simulink model "quadcopter_swarm_Perron_quaternion"  (R2023b)
settings: Solver=ode3  StartTime=0  StopTime=inf  FixedStep=0.005  RelTol=1e-3  EnableMultiTasking=on
values from neighbouring files (symbols this model uses):
  epsilon = 0.24975    [1nrx_dot.mat]    (also in 1nrxdrones_dot.mat; collision_avoidance_POS.mat; collision_avoidance_headonfix_POS.mat; collision_test.mat)
  F_e_g = [0 0 39.28]    [1nrx_dot.mat]    (also in 1nrxdrones_dot.mat; collision_avoidance_POS.mat; collision_avoidance_headonfix_POS.mat; collision_test.mat)
  g = 9.82    [1nrx_dot.mat]    (also in 1nrxdrones_dot.mat; collision_avoidance_POS.mat; collision_avoidance_headonfix_POS.mat; collision_test.mat)
  I_C = [0.5  0  0; 0  0.5  0; 0  0  1]    [1nrx_dot.mat]    (also in 1nrxdrones_dot.mat; collision_avoidance_POS.mat; collision_avoidance_headonfix_POS.mat; collision_test.mat)
  L = [4 -1 -1 -1 -1 0 -1 4 -1 -1 -1 0 ... (36 elements, 6x6)]    [1nrx_dot.mat]    (also in 1nrxdrones_dot.mat; collision_avoidance_POS.mat; collision_avoidance_headonfix_POS.mat; collision_test.mat)
  m = 4    [1nrx_dot.mat]    (also in 1nrxdrones_dot.mat; collision_avoidance_POS.mat; collision_avoidance_headonfix_POS.mat; collision_test.mat)
  M_RB = [4 0 0 0 0 0 0 4 0 0 0 0 ... (36 elements, 6x6)]    [1nrx_dot.mat]    (also in 1nrxdrones_dot.mat; collision_avoidance_POS.mat; collision_avoidance_headonfix_POS.mat; collision_test.mat)
  p_0 = [5  10; 5  -5; -8  5; 5  -13; 8  8; 0  0]    [1nrx_dot.mat]    (also in 1nrxdrones_dot.mat; collision_avoidance_POS.mat; collision_avoidance_headonfix_POS.mat; collision_test.mat)
  p_d = [1  0; 4  0; -2  0; 7  0; 9  0; 0  0]    [1nrx_dot.mat]    (also in 1nrxdrones_dot.mat; collision_avoidance_POS.mat; collision_avoidance_headonfix_POS.mat; collision_test.mat)
  V = [1 2 3 4 5 6]    [1nrx_dot.mat]    (also in 1nrxdrones_dot.mat; collision_avoidance_POS.mat; collision_avoidance_headonfix_POS.mat; collision_test.mat)
undefined symbols (not defined in the file or in its folder): PID_angle_max, PID_inner_max, PID_outer_max, PID_thrust_max
libraries: slpidlib x24, simulink_extras x20, dspsigops x15, sharedtransform x13, aerolibutil x11, dspindex x4, sharedutil x1, vrlib x1
(part 5 of 5)

== system quadcopter_swarm_Perron_quaternion/Master drone/Formatting/Euler to VR/Quaternion Normalization1 ==
  e0 : Inport
  1/2 : Gain  Gain=1/2  SaturateOnIntegerOverflow=on  OutDataTypeStr=Inherit: Same as input  ParamDataTypeStr=Inherit: Same as input
  Demux : Demux  Outputs=[1 3]
      settings: DisplayOption=none
  Mux : Mux  Inputs=2
  Product : Product  InputSameDT=on  SaturateOnIntegerOverflow=on  OutDataTypeStr=Inherit: Same as first input
  Trigonometric Function : Trigonometry
  Trigonometric Function1 : Trigonometry  Operator=cos
  e0_norm : Outport  VectorParamsAs1DForOutWhenUnconnected=off
  wires:
  e0/1 -> Demux/1
  1/2/1 -> Trigonometric Function/1, Trigonometric Function1/1
  Trigonometric Function/1 -> Product/1
  Product/1 -> Mux/2
  Mux/1 -> e0_norm/1
  Demux/1 -> 1/2/1
  Demux/2 -> Product/2
  Trigonometric Function1/1 -> Mux/1

== system quadcopter_swarm_Perron_quaternion/Master drone/Formatting/Euler to VR/Quaternion Normalization2 ==
  e0 : Inport
  1/2 : Gain  Gain=1/2  SaturateOnIntegerOverflow=on  OutDataTypeStr=Inherit: Same as input  ParamDataTypeStr=Inherit: Same as input
  Demux : Demux  Outputs=[1 3]
      settings: DisplayOption=none
  Mux : Mux  Inputs=2
  Product : Product  InputSameDT=on  SaturateOnIntegerOverflow=on  OutDataTypeStr=Inherit: Same as first input
  Trigonometric Function : Trigonometry
  Trigonometric Function1 : Trigonometry  Operator=cos
  e0_norm : Outport  VectorParamsAs1DForOutWhenUnconnected=off
  wires:
  Trigonometric Function1/1 -> Mux/1
  Demux/2 -> Product/2
  Demux/1 -> 1/2/1
  Mux/1 -> e0_norm/1
  Product/1 -> Mux/2
  Trigonometric Function/1 -> Product/1
  1/2/1 -> Trigonometric Function1/1, Trigonometric Function/1
  e0/1 -> Demux/1

== system quadcopter_swarm_Perron_quaternion/Master drone/Quadcopter model Euler/Gravity/euler_to_rotation ==
  eta_euler : Inport
  Rotation Angles to Direction Cosine Matrix : sharedtransform/Rotation Angles to Direction Cosine Matrix  rotationOrder=XYZ  aMode=aMode
  Selector : Selector  InputPortWidth=6  IndexOptions=Index vector (dialog)  Indices=4:6  OutputSizes=1
  R_e_b : Outport
  wires:
  Selector/1 -> Rotation Angles to Direction Cosine Matrix/1  "Theta_0"
  eta_euler/1 -> Selector/1
  Rotation Angles to Direction Cosine Matrix/1 -> R_e_b/1

== system quadcopter_swarm_Perron_quaternion/Master drone2/Formatting/Euler to VR/Axis Angle Vector ==
  e0 : Inport
  2 : Gain  Gain=2  SaturateOnIntegerOverflow=on  OutDataTypeStr=Inherit: Same as input  ParamDataTypeStr=Inherit: Same as input
  Constant : Constant  Value=1e-6
  Demux : Demux  Outputs=[1 3 ]
      settings: DisplayOption=none
  Mux : Mux  Inputs=2
  Product : Product  Inputs=*/  InputSameDT=on  SaturateOnIntegerOverflow=on  OutDataTypeStr=Inherit: Same as first input
  Switch : Switch  Criteria=u2 ~= 0  SaturateOnIntegerOverflow=off  InputSameDT=off
  Trigonometric Function : Trigonometry
  Trigonometric Function2 : Trigonometry  Operator=acos
  e0_norm : Outport  VectorParamsAs1DForOutWhenUnconnected=off
  wires:
  Demux/1 -> Trigonometric Function2/1
  Demux/2 -> Product/1
  Mux/1 -> e0_norm/1
  Product/1 -> Mux/1
  2/1 -> Mux/2
  Trigonometric Function/1 -> Switch/1, Switch/2
  Trigonometric Function2/1 -> Trigonometric Function/1, 2/1
  e0/1 -> Demux/1
  Constant/1 -> Switch/3
  Switch/1 -> Product/2

== system quadcopter_swarm_Perron_quaternion/Master drone2/Formatting/Euler to VR/Quaternion Normalization ==
  e0 : Inport
  1/2 : Gain  Gain=1/2  SaturateOnIntegerOverflow=on  OutDataTypeStr=Inherit: Same as input  ParamDataTypeStr=Inherit: Same as input
  Demux : Demux  Outputs=[1 3]
      settings: DisplayOption=none
  Mux : Mux  Inputs=2
  Product : Product  InputSameDT=on  SaturateOnIntegerOverflow=on  OutDataTypeStr=Inherit: Same as first input
  Trigonometric Function : Trigonometry
  Trigonometric Function1 : Trigonometry  Operator=cos
  e0_norm : Outport  VectorParamsAs1DForOutWhenUnconnected=off
  wires:
  Trigonometric Function1/1 -> Mux/1
  Demux/2 -> Product/2
  Demux/1 -> 1/2/1
  Mux/1 -> e0_norm/1
  Product/1 -> Mux/2
  Trigonometric Function/1 -> Product/1
  1/2/1 -> Trigonometric Function1/1, Trigonometric Function/1
  e0/1 -> Demux/1

== system quadcopter_swarm_Perron_quaternion/Master drone2/Formatting/Euler to VR/Quaternion Normalization1 ==
  e0 : Inport
  1/2 : Gain  Gain=1/2  SaturateOnIntegerOverflow=on  OutDataTypeStr=Inherit: Same as input  ParamDataTypeStr=Inherit: Same as input
  Demux : Demux  Outputs=[1 3]
      settings: DisplayOption=none
  Mux : Mux  Inputs=2
  Product : Product  InputSameDT=on  SaturateOnIntegerOverflow=on  OutDataTypeStr=Inherit: Same as first input
  Trigonometric Function : Trigonometry
  Trigonometric Function1 : Trigonometry  Operator=cos
  e0_norm : Outport  VectorParamsAs1DForOutWhenUnconnected=off
  wires:
  e0/1 -> Demux/1
  1/2/1 -> Trigonometric Function/1, Trigonometric Function1/1
  Trigonometric Function/1 -> Product/1
  Product/1 -> Mux/2
  Mux/1 -> e0_norm/1
  Demux/1 -> 1/2/1
  Demux/2 -> Product/2
  Trigonometric Function1/1 -> Mux/1

== system quadcopter_swarm_Perron_quaternion/Master drone2/Formatting/Euler to VR/Quaternion Normalization2 ==
  e0 : Inport
  1/2 : Gain  Gain=1/2  SaturateOnIntegerOverflow=on  OutDataTypeStr=Inherit: Same as input  ParamDataTypeStr=Inherit: Same as input
  Demux : Demux  Outputs=[1 3]
      settings: DisplayOption=none
  Mux : Mux  Inputs=2
  Product : Product  InputSameDT=on  SaturateOnIntegerOverflow=on  OutDataTypeStr=Inherit: Same as first input
  Trigonometric Function : Trigonometry
  Trigonometric Function1 : Trigonometry  Operator=cos
  e0_norm : Outport  VectorParamsAs1DForOutWhenUnconnected=off
  wires:
  Trigonometric Function1/1 -> Mux/1
  Demux/2 -> Product/2
  Demux/1 -> 1/2/1
  Mux/1 -> e0_norm/1
  Product/1 -> Mux/2
  Trigonometric Function/1 -> Product/1
  1/2/1 -> Trigonometric Function1/1, Trigonometric Function/1
  e0/1 -> Demux/1

== system quadcopter_swarm_Perron_quaternion/Master drone2/Quadcopter model Euler/Gravity/euler_to_rotation ==
  eta_euler : Inport
  Rotation Angles to Direction Cosine Matrix : sharedtransform/Rotation Angles to Direction Cosine Matrix  rotationOrder=XYZ  aMode=aMode
  Selector : Selector  InputPortWidth=6  IndexOptions=Index vector (dialog)  Indices=4:6  OutputSizes=1
  R_e_b : Outport
  wires:
  Selector/1 -> Rotation Angles to Direction Cosine Matrix/1  "Theta_0"
  eta_euler/1 -> Selector/1
  Rotation Angles to Direction Cosine Matrix/1 -> R_e_b/1

== system quadcopter_swarm_Perron_quaternion/Master drone3/Formatting/Euler to VR/Axis Angle Vector ==
  e0 : Inport
  2 : Gain  Gain=2  SaturateOnIntegerOverflow=on  OutDataTypeStr=Inherit: Same as input  ParamDataTypeStr=Inherit: Same as input
  Constant : Constant  Value=1e-6
  Demux : Demux  Outputs=[1 3 ]
      settings: DisplayOption=none
  Mux : Mux  Inputs=2
  Product : Product  Inputs=*/  InputSameDT=on  SaturateOnIntegerOverflow=on  OutDataTypeStr=Inherit: Same as first input
  Switch : Switch  Criteria=u2 ~= 0  SaturateOnIntegerOverflow=off  InputSameDT=off
  Trigonometric Function : Trigonometry
  Trigonometric Function2 : Trigonometry  Operator=acos
  e0_norm : Outport  VectorParamsAs1DForOutWhenUnconnected=off
  wires:
  Demux/1 -> Trigonometric Function2/1
  Demux/2 -> Product/1
  Mux/1 -> e0_norm/1
  Product/1 -> Mux/1
  2/1 -> Mux/2
  Trigonometric Function/1 -> Switch/1, Switch/2
  Trigonometric Function2/1 -> Trigonometric Function/1, 2/1
  e0/1 -> Demux/1
  Constant/1 -> Switch/3
  Switch/1 -> Product/2

== system quadcopter_swarm_Perron_quaternion/Master drone3/Formatting/Euler to VR/Quaternion Normalization ==
  e0 : Inport
  1/2 : Gain  Gain=1/2  SaturateOnIntegerOverflow=on  OutDataTypeStr=Inherit: Same as input  ParamDataTypeStr=Inherit: Same as input
  Demux : Demux  Outputs=[1 3]
      settings: DisplayOption=none
  Mux : Mux  Inputs=2
  Product : Product  InputSameDT=on  SaturateOnIntegerOverflow=on  OutDataTypeStr=Inherit: Same as first input
  Trigonometric Function : Trigonometry
  Trigonometric Function1 : Trigonometry  Operator=cos
  e0_norm : Outport  VectorParamsAs1DForOutWhenUnconnected=off
  wires:
  Trigonometric Function1/1 -> Mux/1
  Demux/2 -> Product/2
  Demux/1 -> 1/2/1
  Mux/1 -> e0_norm/1
  Product/1 -> Mux/2
  Trigonometric Function/1 -> Product/1
  1/2/1 -> Trigonometric Function1/1, Trigonometric Function/1
  e0/1 -> Demux/1

== system quadcopter_swarm_Perron_quaternion/Master drone3/Formatting/Euler to VR/Quaternion Normalization1 ==
  e0 : Inport
  1/2 : Gain  Gain=1/2  SaturateOnIntegerOverflow=on  OutDataTypeStr=Inherit: Same as input  ParamDataTypeStr=Inherit: Same as input
  Demux : Demux  Outputs=[1 3]
      settings: DisplayOption=none
  Mux : Mux  Inputs=2
  Product : Product  InputSameDT=on  SaturateOnIntegerOverflow=on  OutDataTypeStr=Inherit: Same as first input
  Trigonometric Function : Trigonometry
  Trigonometric Function1 : Trigonometry  Operator=cos
  e0_norm : Outport  VectorParamsAs1DForOutWhenUnconnected=off
  wires:
  e0/1 -> Demux/1
  1/2/1 -> Trigonometric Function/1, Trigonometric Function1/1
  Trigonometric Function/1 -> Product/1
  Product/1 -> Mux/2
  Mux/1 -> e0_norm/1
  Demux/1 -> 1/2/1
  Demux/2 -> Product/2
  Trigonometric Function1/1 -> Mux/1

== system quadcopter_swarm_Perron_quaternion/Master drone3/Formatting/Euler to VR/Quaternion Normalization2 ==
  e0 : Inport
  1/2 : Gain  Gain=1/2  SaturateOnIntegerOverflow=on  OutDataTypeStr=Inherit: Same as input  ParamDataTypeStr=Inherit: Same as input
  Demux : Demux  Outputs=[1 3]
      settings: DisplayOption=none
  Mux : Mux  Inputs=2
  Product : Product  InputSameDT=on  SaturateOnIntegerOverflow=on  OutDataTypeStr=Inherit: Same as first input
  Trigonometric Function : Trigonometry
  Trigonometric Function1 : Trigonometry  Operator=cos
  e0_norm : Outport  VectorParamsAs1DForOutWhenUnconnected=off
  wires:
  Trigonometric Function1/1 -> Mux/1
  Demux/2 -> Product/2
  Demux/1 -> 1/2/1
  Mux/1 -> e0_norm/1
  Product/1 -> Mux/2
  Trigonometric Function/1 -> Product/1
  1/2/1 -> Trigonometric Function1/1, Trigonometric Function/1
  e0/1 -> Demux/1

== system quadcopter_swarm_Perron_quaternion/Master drone3/Quadcopter model Euler/Gravity/euler_to_rotation ==
  eta_euler : Inport
  Rotation Angles to Direction Cosine Matrix : sharedtransform/Rotation Angles to Direction Cosine Matrix  rotationOrder=XYZ  aMode=aMode
  Selector : Selector  InputPortWidth=6  IndexOptions=Index vector (dialog)  Indices=4:6  OutputSizes=1
  R_e_b : Outport
  wires:
  Selector/1 -> Rotation Angles to Direction Cosine Matrix/1  "Theta_0"
  eta_euler/1 -> Selector/1
  Rotation Angles to Direction Cosine Matrix/1 -> R_e_b/1

== system quadcopter_swarm_Perron_quaternion/Master drone4/Formatting/Euler to VR/Axis Angle Vector ==
  e0 : Inport
  2 : Gain  Gain=2  SaturateOnIntegerOverflow=on  OutDataTypeStr=Inherit: Same as input  ParamDataTypeStr=Inherit: Same as input
  Constant : Constant  Value=1e-6
  Demux : Demux  Outputs=[1 3 ]
      settings: DisplayOption=none
  Mux : Mux  Inputs=2
  Product : Product  Inputs=*/  InputSameDT=on  SaturateOnIntegerOverflow=on  OutDataTypeStr=Inherit: Same as first input
  Switch : Switch  Criteria=u2 ~= 0  SaturateOnIntegerOverflow=off  InputSameDT=off
  Trigonometric Function : Trigonometry
  Trigonometric Function2 : Trigonometry  Operator=acos
  e0_norm : Outport  VectorParamsAs1DForOutWhenUnconnected=off
  wires:
  Demux/1 -> Trigonometric Function2/1
  Demux/2 -> Product/1
  Mux/1 -> e0_norm/1
  Product/1 -> Mux/1
  2/1 -> Mux/2
  Trigonometric Function/1 -> Switch/1, Switch/2
  Trigonometric Function2/1 -> Trigonometric Function/1, 2/1
  e0/1 -> Demux/1
  Constant/1 -> Switch/3
  Switch/1 -> Product/2

== system quadcopter_swarm_Perron_quaternion/Master drone4/Formatting/Euler to VR/Quaternion Normalization ==
  e0 : Inport
  1/2 : Gain  Gain=1/2  SaturateOnIntegerOverflow=on  OutDataTypeStr=Inherit: Same as input  ParamDataTypeStr=Inherit: Same as input
  Demux : Demux  Outputs=[1 3]
      settings: DisplayOption=none
  Mux : Mux  Inputs=2
  Product : Product  InputSameDT=on  SaturateOnIntegerOverflow=on  OutDataTypeStr=Inherit: Same as first input
  Trigonometric Function : Trigonometry
  Trigonometric Function1 : Trigonometry  Operator=cos
  e0_norm : Outport  VectorParamsAs1DForOutWhenUnconnected=off
  wires:
  Trigonometric Function1/1 -> Mux/1
  Demux/2 -> Product/2
  Demux/1 -> 1/2/1
  Mux/1 -> e0_norm/1
  Product/1 -> Mux/2
  Trigonometric Function/1 -> Product/1
  1/2/1 -> Trigonometric Function1/1, Trigonometric Function/1
  e0/1 -> Demux/1

== system quadcopter_swarm_Perron_quaternion/Master drone4/Formatting/Euler to VR/Quaternion Normalization1 ==
  e0 : Inport
  1/2 : Gain  Gain=1/2  SaturateOnIntegerOverflow=on  OutDataTypeStr=Inherit: Same as input  ParamDataTypeStr=Inherit: Same as input
  Demux : Demux  Outputs=[1 3]
      settings: DisplayOption=none
  Mux : Mux  Inputs=2
  Product : Product  InputSameDT=on  SaturateOnIntegerOverflow=on  OutDataTypeStr=Inherit: Same as first input
  Trigonometric Function : Trigonometry
  Trigonometric Function1 : Trigonometry  Operator=cos
  e0_norm : Outport  VectorParamsAs1DForOutWhenUnconnected=off
  wires:
  e0/1 -> Demux/1
  1/2/1 -> Trigonometric Function/1, Trigonometric Function1/1
  Trigonometric Function/1 -> Product/1
  Product/1 -> Mux/2
  Mux/1 -> e0_norm/1
  Demux/1 -> 1/2/1
  Demux/2 -> Product/2
  Trigonometric Function1/1 -> Mux/1

== system quadcopter_swarm_Perron_quaternion/Master drone4/Formatting/Euler to VR/Quaternion Normalization2 ==
  e0 : Inport
  1/2 : Gain  Gain=1/2  SaturateOnIntegerOverflow=on  OutDataTypeStr=Inherit: Same as input  ParamDataTypeStr=Inherit: Same as input
  Demux : Demux  Outputs=[1 3]
      settings: DisplayOption=none
  Mux : Mux  Inputs=2
  Product : Product  InputSameDT=on  SaturateOnIntegerOverflow=on  OutDataTypeStr=Inherit: Same as first input
  Trigonometric Function : Trigonometry
  Trigonometric Function1 : Trigonometry  Operator=cos
  e0_norm : Outport  VectorParamsAs1DForOutWhenUnconnected=off
  wires:
  Trigonometric Function1/1 -> Mux/1
  Demux/2 -> Product/2
  Demux/1 -> 1/2/1
  Mux/1 -> e0_norm/1
  Product/1 -> Mux/2
  Trigonometric Function/1 -> Product/1
  1/2/1 -> Trigonometric Function1/1, Trigonometric Function/1
  e0/1 -> Demux/1

== matlab function quadcopter_swarm_Perron_quaternion/Master drone/Quadcopter model Euler/rigid-body dynamics/MATLAB Function ==
  data: tau input; nu_dot output; nu input; I_C input; M_RB input; m input
function nu_dot = fcn(tau,nu,I_C,M_RB,m)

omega_b_b_e = nu(4:6);

C_RB = [
    m*skew_sym(omega_b_b_e)     zeros(3)
    zeros(3)                    -skew_sym(I_C*omega_b_b_e)
];

nu_dot = inv(M_RB)*(tau - C_RB*nu);

end


function res = skew_sym(vector)

res = [
    0               -vector(3)      vector(2)
    vector(3)       0               -vector(1)
    -vector(2)     vector(1)       0
];

end

== matlab function quadcopter_swarm_Perron_quaternion/Master drone2/PID controllers/outer-loop position controller/MATLAB Function1 ==
  data: Deltap_e input; Deltap_b output; psi input
function Deltap_b = fcn(Deltap_e,psi)

R = [ cos(psi) , -sin(psi) ;
      sin(psi) ,  cos(psi) ];

Deltap_b = R'*Deltap_e;

== matlab function quadcopter_swarm_Perron_quaternion/Master drone2/Quadcopter model Euler/kinematics from Euler angles/MATLAB Function1 ==
  data: eta input; nu input; eta_dot output
function eta_dot = fcn(eta, nu)

% Get angles
phi = eta(4);
theta = eta(5);
psi = eta(6);

% Get R_e_b_Theta

% yaw
R_z = [ 
    cos(psi)    -sin(psi)   0
    sin(psi)    cos(psi)    0
    0           0           1
];

% pitch
R_y = [
    cos(theta)  0           sin(theta)
    0           1           0
    -sin(theta) 0           cos(theta)
];

% roll
R_x = [
    1           0           0
    0           cos(phi)    -sin(phi)
    0           sin(phi)    cos(phi)
];

% result
R_be = R_z*R_y*R_x;

% Get T_Theta

T_Theta = [
    1       sin(phi)*tan(theta)     cos(phi)*tan(theta)
    0       cos(phi)                -sin(phi)
    0       sin(phi)/cos(theta)     cos(phi)/cos(theta)
];

% Get J_Theta

J_Theta = [
    R_be     zeros(3)
    zeros(3)        T_Theta
];

eta_dot = J_Theta*nu;

end

== matlab function quadcopter_swarm_Perron_quaternion/Master drone2/Quadcopter model Euler/rigid-body dynamics/MATLAB Function ==
  data: tau input; nu_dot output; nu input; I_C input; M_RB input; m input
function nu_dot = fcn(tau,nu,I_C,M_RB,m)

omega_b_b_e = nu(4:6);

C_RB = [
    m*skew_sym(omega_b_b_e)     zeros(3)
    zeros(3)                    -skew_sym(I_C*omega_b_b_e)
];

nu_dot = inv(M_RB)*(tau - C_RB*nu);

end


function res = skew_sym(vector)

res = [
    0               -vector(3)      vector(2)
    vector(3)       0               -vector(1)
    -vector(2)     vector(1)       0
];

end

== matlab function quadcopter_swarm_Perron_quaternion/Master drone3/PID controllers/outer-loop position controller/MATLAB Function1 ==
  data: Deltap_e input; Deltap_b output; psi input
function Deltap_b = fcn(Deltap_e,psi)

R = [ cos(psi) , -sin(psi) ;
      sin(psi) ,  cos(psi) ];

Deltap_b = R'*Deltap_e;

== matlab function quadcopter_swarm_Perron_quaternion/Master drone3/Quadcopter model Euler/kinematics from Euler angles/MATLAB Function1 ==
  data: eta input; nu input; eta_dot output
function eta_dot = fcn(eta, nu)

% Get angles
phi = eta(4);
theta = eta(5);
psi = eta(6);

% Get R_e_b_Theta

% yaw
R_z = [ 
    cos(psi)    -sin(psi)   0
    sin(psi)    cos(psi)    0
    0           0           1
];

% pitch
R_y = [
    cos(theta)  0           sin(theta)
    0           1           0
    -sin(theta) 0           cos(theta)
];

% roll
R_x = [
    1           0           0
    0           cos(phi)    -sin(phi)
    0           sin(phi)    cos(phi)
];

% result
R_be = R_z*R_y*R_x;

% Get T_Theta

T_Theta = [
    1       sin(phi)*tan(theta)     cos(phi)*tan(theta)
    0       cos(phi)                -sin(phi)
    0       sin(phi)/cos(theta)     cos(phi)/cos(theta)
];

% Get J_Theta

J_Theta = [
    R_be     zeros(3)
    zeros(3)        T_Theta
];

eta_dot = J_Theta*nu;

end

== matlab function quadcopter_swarm_Perron_quaternion/Master drone3/Quadcopter model Euler/rigid-body dynamics/MATLAB Function ==
  data: tau input; nu_dot output; nu input; I_C input; M_RB input; m input
function nu_dot = fcn(tau,nu,I_C,M_RB,m)

omega_b_b_e = nu(4:6);

C_RB = [
    m*skew_sym(omega_b_b_e)     zeros(3)
    zeros(3)                    -skew_sym(I_C*omega_b_b_e)
];

nu_dot = inv(M_RB)*(tau - C_RB*nu);

end


function res = skew_sym(vector)

res = [
    0               -vector(3)      vector(2)
    vector(3)       0               -vector(1)
    -vector(2)     vector(1)       0
];

end

== matlab function quadcopter_swarm_Perron_quaternion/Master drone4/PID controllers/outer-loop position controller/MATLAB Function1 ==
  data: Deltap_e input; Deltap_b output; psi input
function Deltap_b = fcn(Deltap_e,psi)

R = [ cos(psi) , -sin(psi) ;
      sin(psi) ,  cos(psi) ];

Deltap_b = R'*Deltap_e;

== matlab function quadcopter_swarm_Perron_quaternion/Master drone4/Quadcopter model/rigid-body dynamics/MATLAB Function ==
  data: tau input; nu_dot output; nu input; I_C input; M_RB input; m input
function nu_dot = fcn(tau,nu,I_C,M_RB,m)

omega_b_b_e = nu(4:6);

C_RB = [
    m*skew_sym(omega_b_b_e)     zeros(3)
    zeros(3)                    -skew_sym(I_C*omega_b_b_e)
];

nu_dot = inv(M_RB)*(tau - C_RB*nu);

end


function res = skew_sym(vector)

res = [
    0               -vector(3)      vector(2)
    vector(3)       0               -vector(1)
    -vector(2)     vector(1)       0
];

end

== matlab function quadcopter_swarm_Perron_quaternion/Master drone/PID controllers/outer-loop position controller/MATLAB Function1 ==
  data: Deltap_e input; Deltap_b output; psi input
function Deltap_b = fcn(Deltap_e,psi)

R = [ cos(psi) , -sin(psi) ;
      sin(psi) ,  cos(psi) ];

Deltap_b = R'*Deltap_e;

== matlab function quadcopter_swarm_Perron_quaternion/Master drone/Quadcopter model Euler/kinematics from Euler angles/MATLAB Function1 ==
  data: eta input; nu input; eta_dot output
function eta_dot = fcn(eta, nu)

% Get angles
phi = eta(4);
theta = eta(5);
psi = eta(6);

% Get R_e_b_Theta

% yaw
R_z = [ 
    cos(psi)    -sin(psi)   0
    sin(psi)    cos(psi)    0
    0           0           1
];

% pitch
R_y = [
    cos(theta)  0           sin(theta)
    0           1           0
    -sin(theta) 0           cos(theta)
];

% roll
R_x = [
    1           0           0
    0           cos(phi)    -sin(phi)
    0           sin(phi)    cos(phi)
];

% result
R_be = R_z*R_y*R_x;

% Get T_Theta

T_Theta = [
    1       sin(phi)*tan(theta)     cos(phi)*tan(theta)
    0       cos(phi)                -sin(phi)
    0       sin(phi)/cos(theta)     cos(phi)/cos(theta)
];

% Get J_Theta

J_Theta = [
    R_be     zeros(3)
    zeros(3)        T_Theta
];

eta_dot = J_Theta*nu;

end
